simulink model "RRpendulum_digtwin"  (R2025b)
settings: Solver=FixedStepAuto  StartTime=0.0  StopTime=inf  FixedStep=0.001  RelTol=1e-3  EnableMultiTasking=on
PreLoadFcn:
  | %define mechanical pars, init conditions
  | run RRpendulum_Parameters_num.m
  | 
  | %% parameters moved to model workspace
  | % sample time
  | %T_SAMPLE = 0.001;
  | 
  | %microsteps per turn of 200 step motor @ x16 microstepping
  | %STEPS_PER_TURN = 3200;
  | 
  | %encoder counts per turn
  | %COUNTS_PER_TURN = 2400;
model workspace (MAT data in the model file):
  COUNTS_PER_TURN = 2400
  STEPS_PER_TURN = 3200
  T_SAMPLE = 0.001
undefined symbols (not defined in the file): g_num, l_num, m_num, r_num
libraries: digtwin_labo_lib x1
(part 2 of 2)

== stateflow chart RRpendulum_digtwin/Controller ==
  settings: updateMethod=DISCRETE  sampleTime=T_SAMPLE
  state Startup
    accel_cmd = 2*pi/3200; % to get 1 step/s^2
  state Startup1
    accel_cmd = 0;
  state Swingup
    en:
    accelpulseampl = 30; %rad/s
    accelpulsetime = 0.1; %s
    du:
    accel_cmd = 0;
    state accelposstart
      en,du:
      accel_cmd = accelpulseampl;
    state decelnegstart
      en,du:
      accel_cmd = -1*accelpulseampl;
    state stoppedpos
    state stoppedpos1
    (default) -> accelposstart
    accelposstart -> decelnegstart : after(accelpulsetime,sec)
    decelnegstart -> stoppedpos : after(accelpulsetime,sec)
    stoppedpos -> stoppedpos1
  state Stabilize
    en:
    if (abs(pi-states(3)) < abs(-pi-states(3)))
    ref_state = [0;0;pi;0];
    else
    ref_state = [0;0;-pi;0];
    end
    en,du:
    accel_cmd=K*(ref_state-states);
  (default) -> Startup
  Startup -> Startup1
  Startup1 -> Swingup : after(.2,sec)
  Swingup -> Stabilize : [abs(abs(states(3))-pi)<epsilon]
  data: Etot input; Ekin input; Epot input; accel_cmd output size=1; states input; K parameter; epsilon parameter; g_num parameter; m_num parameter; r_num parameter; l_num parameter; Etgt local; deadzone local; stiffness local; accelpulseampl local; accelpulsetime local; q2zcpos input; q2zcneg input; q2pkneg input; q2pkpos input; ref_state local

== matlab function RRpendulum_digtwin/MATLAB Function ==
  data: Etot output; Ekin output; Epot output; states input; g_num parameter; m_num parameter; r_num parameter; l_num parameter
function [Etot,Ekin,Epot]=calc_energy(states, g_num, m_num, r_num, l_num)
%q1=states(1);
v1=states(2);
q2=states(3);
v2=states(4);

Ekin=l_num^2*m_num*(v1^2 + v2^2)/2 + m_num*r_num^2*v1^2/2 - l_num^2*m_num*cos(q2)^2*v1^2/2 + l_num*m_num*r_num*cos(q2)*v2*v1;
Epot = -g_num*l_num*m_num*cos(q2)+m_num*g_num*l_num;
Etot = Ekin+Epot;
